simulink model "level11"  (R2017a)
settings: Solver=VariableStepAuto  StartTime=0.0  StopTime=0.5  MaxStep=1e-4  RelTol=1e-3
libraries: simulink x5, powerlib x4, powerlib_meascontrol x1
settings Model: Creator=Bilal Ahmed  LastModifiedBy=Bilal Ahmed

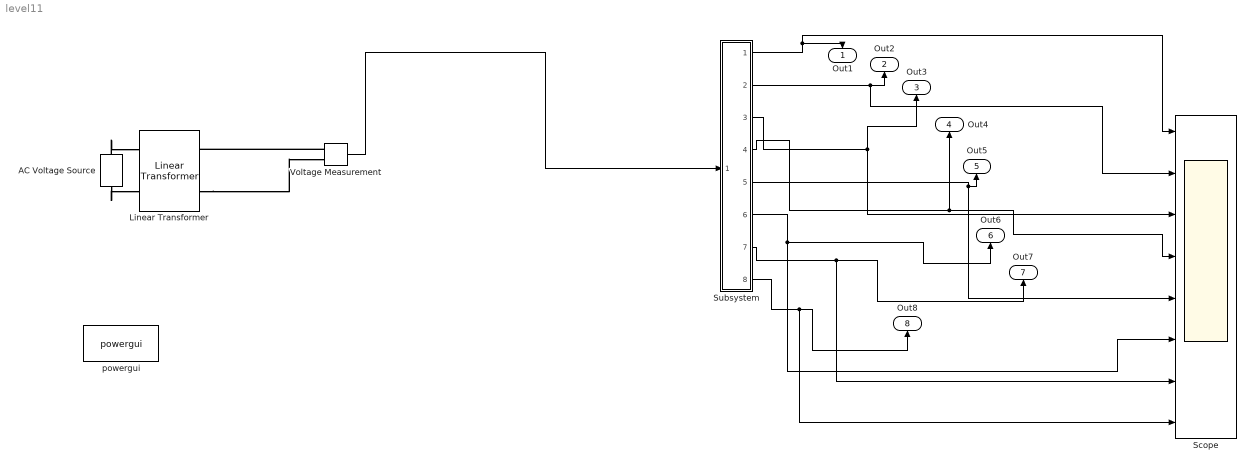
== system level11 ==
  AC Voltage Source : powerlib/Electrical Sources/AC Voltage Source  Amplitude=220  Phase=0  Frequency=50  SampleTime=0  Measurements=None  BusType=PV  Pref=10e3  Qref=0  Qmin=-inf  Qmax=+inf
  Linear Transformer : powerlib/Elements/Linear Transformer  UNITS=pu  NominalPower=[1100 50 ]  winding1=[154 0 0]  winding2=[3.5 0 0]  ThreeWindings=off  winding3=[3.15e+05 9.68e-09 3.2267e-07]  RmLm=[Inf Inf]  Measurements=None  DataType=off
  Scope : Scope  NumInputPorts=8
  Subsystem : Subsystem
  Voltage Measurement : powerlib/Measurements/Voltage Measurement  PhasorSimulation=off  OutputType=Complex  PSBequivalent=0
  powergui : powerlib/powergui  Priority=1  SimulationMode=Continuous  SampleTime=50e-6  frequency=60  Iterations=50  frequencyindice=50  Pbase=100e6  ErrMax=1e-4  UnitsV=kV  UnitsW=MW  buscounter=0  FunctionMessages=off  echomessages=off  EnableUseOfTLC=off  CurrentSourceSwitches=off  DisableSnubberDevices=off  DisableRonSwitches=off  DisableVfSwitches=off  DisplayEquations=off  SolverType=Tustin/Backward Euler (TBE)  Interpol=off  ExternalGateDelay=off  methode=off  Ts=100  x0status=blocks  SPID=on  SwTol=0  HookPort=off  RestoreLinks=warning  ResistiveCurrentMeasurement=off  Frange=[0:2:500]  Ylog=off  Xlog=on  ShowGrid=off  save=off  variable=ZData  structure=0  ZoomFFT=off  StartTime=0.0  cycles=1  DisplayStyle=1  fundamental=60  FreqAxis=off  MaxFrequency=1000  frequencyindicesteady=1  RmsSteady=1  display=off
  Out1 : Outport
  Out2 : Outport  Port=2
  Out3 : Outport  Port=3
  Out4 : Outport  Port=4
  Out5 : Outport  Port=5
  Out6 : Outport  Port=6
  Out7 : Outport  Port=7
  Out8 : Outport  Port=8
  wires:
  Subsystem/4(Out5) -> Scope/4, Out4/1
  Subsystem/6(Out4) -> Scope/6, Out6/1
  Subsystem/7(Out7) -> Scope/7, Out7/1
  Subsystem/8(Out8) -> Scope/8, Out8/1
  Subsystem/5(Out6) -> Scope/5, Out5/1
  Voltage Measurement/1 -> Subsystem/1(In1)
  Subsystem/1(Out1) -> Scope/1, Out1/1
  Subsystem/3(Out3) -> Out3/1, Scope/3
  Subsystem/2(Out2) -> Scope/2, Out2/1
  connections:
  Linear Transformer/RConn2 -- Voltage Measurement/LConn2
  AC Voltage Source/RConn1 -- Linear Transformer/LConn1
  AC Voltage Source/LConn1 -- Linear Transformer/LConn2
  Voltage Measurement/LConn1 -- Linear Transformer/RConn1

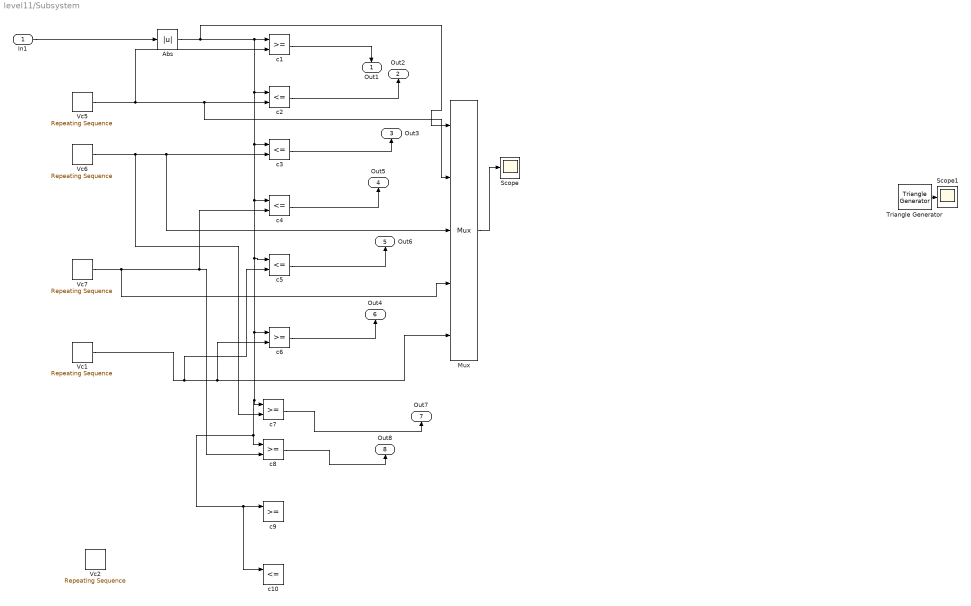
== system level11/Subsystem ==
  In1 : Inport
  Abs : Abs
  Mux : Mux  Inputs=5
  Scope : Scope
  Scope1 : Scope
  Triangle Generator : powerlib_meascontrol/Pulse & Signal Generators/Triangle Generator  Freq=1e6  Phase=0  Ts=0
  Vc1 : simulink/Sources/Repeating Sequence  rep_seq_t=[0 0.00001/2 0.00001]  rep_seq_y=[0 1.25 0]
  Vc2 : simulink/Sources/Repeating Sequence  rep_seq_t=[0 0.00001/2 0.00001]  rep_seq_y=[0 1.25 0]
  Vc5 : simulink/Sources/Repeating Sequence  rep_seq_t=[0 0.00001/2 0.00001]  rep_seq_y=[3.75 5.00 3.75]
  Vc6 : simulink/Sources/Repeating Sequence  rep_seq_t=[0 0.00001/2 0.00001]  rep_seq_y=[2.50 3.75 2.50]
  Vc7 : simulink/Sources/Repeating Sequence  rep_seq_t=[0 0.00001/2 0.00001]  rep_seq_y=[1.25 2.50 1.25]
  c{1,6..9} (5 alike) : RelationalOperator  OutDataTypeStr=boolean  RndMeth=Nearest
  c{2..5,10} (5 alike) : RelationalOperator  Operator=<=  OutDataTypeStr=boolean  RndMeth=Nearest
  Out1 : Outport
  Out2 : Outport  Port=2
  Out3 : Outport  Port=3
  Out5 : Outport  Port=4
  Out6 : Outport  Port=5
  Out4 : Outport  Port=6
  Out7 : Outport  Port=7
  Out8 : Outport  Port=8
  wires:
  c5/1 -> Out6/1
  c6/1 -> Out4/1
  c4/1 -> Out5/1
  c2/1 -> Out2/1
  c1/1 -> Out1/1
  Vc7/1 -> Mux/4, c8/2, c4/2
  Vc5/1 -> c1/2, Mux/2, c2/2
  Vc6/1 -> c7/2, Mux/3, c3/2
  Mux/1 -> Scope/1
  c3/1 -> Out3/1
  Abs/1 -> Mux/1, c2/1, c5/1, c6/1, c10/1, c9/1, c8/1, c7/1, c4/1, c3/1, c1/1
  In1/1 -> Abs/1
  Vc1/1 -> c5/2, c6/2, Mux/5
  c7/1 -> Out7/1
  c8/1 -> Out8/1
  Triangle Generator/1 -> Scope1/1
